simulink model "saturate_rwa_lib_test"  (R2018b)
settings: Solver=VariableStepAuto  StartTime=0.0  StopTime=10.0  RelTol=1e-3
undefined symbols (not defined in the file or in its folder): fswParams
libraries: saturate_rwa_lib x1
settings Model: Creator=taylorreynolds  LastModifiedBy=taylorreynolds

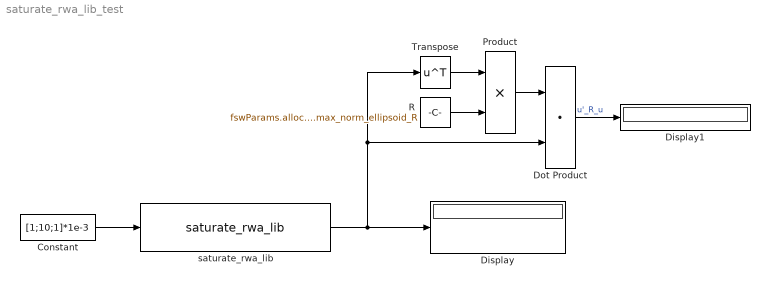
== system saturate_rwa_lib_test ==
  Constant : Constant  Value=[1;10;1]*1e-3
  Display : Display
      settings: Format=long_e
  Display1 : Display
      settings: Format=long_e
  Dot Product : DotProduct  InputSameDT=on  OutDataTypeStr=Inherit: Inherit via internal rule
  Product : Product
  R : Constant  Value=fswParams.allocator.rwa.max_norm_ellipsoid_R
  Transpose : Math  Operator=transpose  SaturateOnIntegerOverflow=on
  saturate_rwa_lib : saturate_rwa_lib/saturate_rwa_lib  SystemSampleTime=-1
  wires:
  Constant/1 -> saturate_rwa_lib/1
  Transpose/1 -> Product/1
  Product/1 -> Dot Product/1
  R/1 -> Product/2
  saturate_rwa_lib/1 -> Dot Product/2, Transpose/1, Display/1
  Dot Product/1 -> Display1/1  "u'_R_u"
